simulink model "om2"  (Simulink 7.2)
settings: Solver=ode45  StartTime=0.0  StopTime=10.0  RelTol=1e-3
libraries: cdsFilt x118, cdsEpicsOut x38, cdsIPC x23, cdsMatrix x10, cdsOsc x8, cdsPhaseDeg x8, cdsEpicsIn x8, cdsRms x8, cdsProduct x5, simulink x2, cdsWD x2, cdsIPCS x1
(part 1 of 6)
settings Model: Creator=Rolf  LastModifiedBy=aivanov  ExtModeAutoUpdateStatusClock=off
settings OptimizationCC: InitFltsAndDblsToZero=on

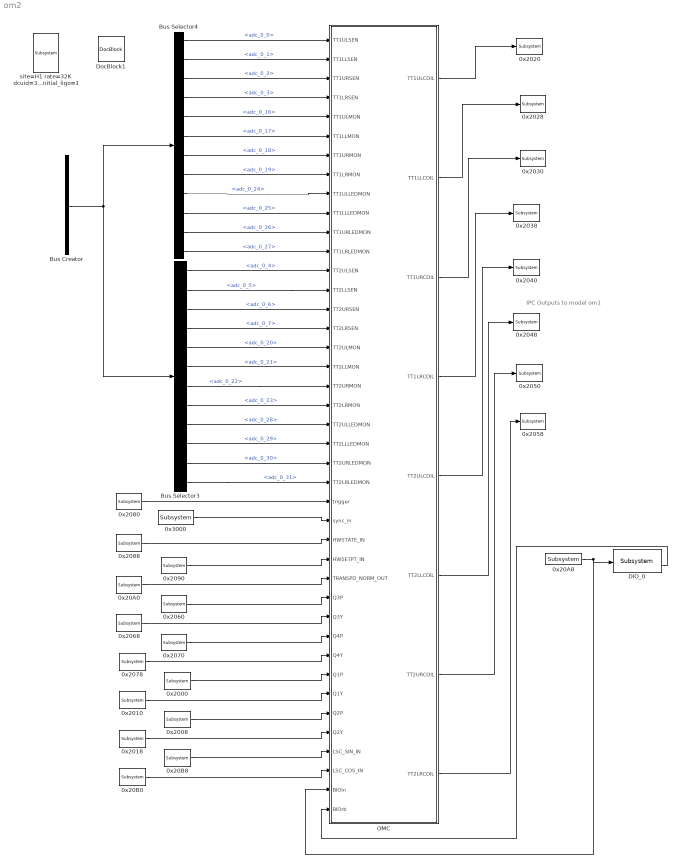
== system om2 ==
  note: IPC Outputs to model om1
  0x{2000,2008,2010,2018,2020,2028,2030,2038,2040,2048,2050,2058,2060,2068,2070,2078,2080,2088,2090} (19 alike) : cdsIPC/Subsystem  Tag=cdsIPC  Description=Inter-process communication through /rtl_epics_ipc shared memory  SystemSampleTime=-1
      settings: AttributesFormatString=%<Tag>
  0x20A0 : cdsIPC/Subsystem  Tag=cdsIPC  Description=Inter-process communication through /rtl_epics_ipc shared memory  SystemSampleTime=-1
      settings: AttributesFormatString=%<Tag>
  0x20A8 : cdsIPC/Subsystem  Tag=cdsIPC  Description=Inter-process communication through /rtl_epics_ipc shared memory  SystemSampleTime=-1
      settings: AttributesFormatString=%<Tag>
  0x20B0 : cdsIPC/Subsystem  Tag=cdsIPC  Description=Inter-process communication through /rtl_epics_ipc shared memory  SystemSampleTime=-1
      settings: AttributesFormatString=%<Tag>
  0x20B8 : cdsIPC/Subsystem  Tag=cdsIPC  Description=Inter-process communication through /rtl_epics_ipc shared memory  SystemSampleTime=-1
      settings: AttributesFormatString=%<Tag>
  0x3000 : cdsIPCS/Subsystem  Tag=cdsIPCS  SystemSampleTime=-1
      settings: AttributesFormatString=%<Tag>
  Bus Creator : BusCreator  Tag=adc_0  Description=|  Inputs='adc_0_0','adc_0_1','adc_0_2','adc_0_3','adc_0_4','adc_0_5','adc_0_6','adc_0_7','adc_0_8','adc_0_9','adc_0_10','adc_0_11','adc_0_12','adc_0_13','adc_0_14','adc_0_15','adc_0_16','adc_0_17','adc_0_18','adc_0_19','adc_0_20','adc_0_21','adc_0_22','adc_0_23','adc_0_24','adc_0_25','adc_0_26','adc_0_27','adc_0_28','adc_0_29','adc_0_30','adc_0_31'
      | PCI66-16AI64SSA
      | 40Vp-p, 16-bit, 610uV/count
      settings: AttributesFormatString=%<Description>\n%<Tag>
  Bus Selector3 : BusSelector  OutputSignals=adc_0_4,adc_0_5,adc_0_6,adc_0_7,adc_0_20,adc_0_21,adc_0_22,adc_0_23,adc_0_28,adc_0_29,adc_0_30,adc_0_31
  Bus Selector4 : BusSelector  OutputSignals=adc_0_0,adc_0_1,adc_0_2,adc_0_3,adc_0_16,adc_0_17,adc_0_18,adc_0_19,adc_0_24,adc_0_25,adc_0_26,adc_0_27
  DIO_0 : cdsRio/Subsystem  Tag=cdsRio  Description=PCI IIRO 8 relay output and isolated input module  SystemSampleTime=-1
      settings: AttributesFormatString=%<Tag>
  DocBlock1 : simulink/Model-Wide Utilities/DocBlock  Tag=SW Install  SystemSampleTime=-1  DocumentType=Text
      content=|
      | *******************************************************
      | Software installation on new computer
      | *******************************************************
      |
      | 1. Install network and PCIe cards.
      |     - Remove top cover and I/O cage.
      |     - Install NIC in PCI-X slot.
      |     - Install PCIe card for I/O chassis in PCIe slot.
      |     - Reinstall I/O cage.
      |     - Close cover.
      | 2. Connect Infiniband cables to I/O chassis and power up I/O chassis.
      | 3. Power up computer.
      | 4. Change root password.
      | 5. Modify network startup.
      |     - edit /etc/sysconfig/network-scripts (can remove all except eth0)
      |     - Change hostname in /etc/sysconfig/network file
      |     - Modify /etc/hosts
      | 6. Add users
      | 7. Make rtLinux
      |     - cd to kernel directory
      |     - Type 'make modules-install install
      |     - Edit /etc/grub_conf and change default to 0 to boot rtLinux on powerup.
      | 8. Get rid of unnecessary tasks.
      |     - cpuspeed
      |     - bluetooth
      |     - avahi daemon
      |     - cups
      |     - cups config
      |     - httpd
      |     - haldaemon
      |     - hidd
      |     - iptables
      |     - isdn
      |     - kudsu
      |     - sendmail
      |     - smartd
      |     - xfs
      | 9. reboot
      | 10. Use del key to bring up boot configuration and get rid of all unnecessary support, such as:
      |     - parallel, serial ports
      |     - USB
      | 11. Install CDS EPICS files
      |     - cd to /opt
      |     - load CDS CD (mount /dev/cdrom /mnt)
      |     - Run 'tar zxf /mnt/epics.tar.gz'
      | 12. Edit /etc/rc.local file and add:
      |     - /opt/rtlinux_dir/rtlinuxpro/mdoules/rtcore&
      |     - /opt/epics-3.14.7-linux/base/bin/linux-x86/caRepeater&
      |     - sleep 5
      |     - /etc/setup_shmem.rtl&
      | 13. Add EPICS libraries to all paths
      |     - cd to /etc/ld.so.conf.d
      |     - edit epics.conf
      |     - Add the following lines to this file:
      |         - /opt/epics-3.14.7-linux/base/lib/linux-x86
      |         - /opt/epics-3.14.7-linux/seq/lib/linux-x86
      | 14. Add CDS source code.
      |     - cd to /home/user
      |     - tar zxf /mnt/cds.tar.gz
      | 15. Build the shmem module.
      |     - cd to /home/user/cds/advLigo/src/fe/shmem
      |     - Type 'make'
      |     - cp shmem.rtl file to /etc
      | 16. Run the rc local file.
      |     - /etc/rc.local
      | 17. Create the gm files.
      |     - untar gm files in root home directory.
      |     - Type make.
      |     - Go to gm binary directory.
      |     - mkdir /opt/gm
      |     - ./GM_INSTALL
      |     - chkconfig --add gm
      |     - chkconfig gm on
      |     - service gm start
      | 18. Need to get rid of possible errors in running sequences looking for caRepeater.
      |     - ln -s /bin/true /bin/caRepeater
      | 19. Reboot
      |
      | ******* Should now be able to build FE code and EPICS.
      settings: AttributesFormatString=%<Tag>
  OMC : Subsystem  Tag=top_names
      settings: AttributesFormatString=%<Tag>
  site=H1 rate=32K dcuid=31 gds_node_id=5 no_sync=1 specific_cpu=2 compat_initial_ligo=1 : cdsParameters/Subsystem  Tag=cdsParameters  SystemSampleTime=-1
      settings: AttributesFormatString=%<Tag>
  wires:
  Bus Creator/1 -> Bus Selector4/1, Bus Selector3/1
  Bus Selector4/1 -> OMC/1(TT1ULSEN)  "<adc_0_0>"
  Bus Selector4/2 -> OMC/2(TT1LLSEN)  "<adc_0_1>"
  Bus Selector4/3 -> OMC/3(TT1URSEN)  "<adc_0_2>"
  Bus Selector4/4 -> OMC/4(TT1LRSEN)  "<adc_0_3>"
  Bus Selector4/5 -> OMC/5(TT1ULMON)  "<adc_0_16>"
  Bus Selector4/6 -> OMC/6(TT1LLMON)  "<adc_0_17>"
  Bus Selector4/7 -> OMC/7(TT1URMON)  "<adc_0_18>"
  Bus Selector4/8 -> OMC/8(TT1LRMON)  "<adc_0_19>"
  Bus Selector4/9 -> OMC/9(TT1ULLEDMON)  "<adc_0_24>"
  Bus Selector4/10 -> OMC/10(TT1LLLEDMON)  "<adc_0_25>"
  Bus Selector4/11 -> OMC/11(TT1URLEDMON)  "<adc_0_26>"
  Bus Selector4/12 -> OMC/12(TT1LRLEDMON)  "<adc_0_27>"
  Bus Selector3/1 -> OMC/13(TT2ULSEN)  "<adc_0_4>"
  Bus Selector3/2 -> OMC/14(TT2LLSEN)  "<adc_0_5>"
  Bus Selector3/4 -> OMC/16(TT2LRSEN)  "<adc_0_7>"
  Bus Selector3/5 -> OMC/17(TT2ULMON)  "<adc_0_20>"
  Bus Selector3/7 -> OMC/19(TT2URMON)  "<adc_0_22>"
  Bus Selector3/8 -> OMC/20(TT2LRMON)  "<adc_0_23>"
  Bus Selector3/9 -> OMC/21(TT2ULLEDMON)  "<adc_0_28>"
  Bus Selector3/10 -> OMC/22(TT2LLLEDMON)  "<adc_0_29>"
  Bus Selector3/11 -> OMC/23(TT2URLEDMON)  "<adc_0_30>"
  Bus Selector3/12 -> OMC/24(TT2LRLEDMON)  "<adc_0_31>"
  OMC/1(TT1ULCOIL) -> 0x2020/1
  OMC/2(TT1LLCOIL) -> 0x2028/1
  OMC/3(TT1URCOIL) -> 0x2030/1
  OMC/4(TT1LRCOIL) -> 0x2038/1
  OMC/5(TT2ULCOIL) -> 0x2040/1
  OMC/6(TT2LLCOIL) -> 0x2048/1
  OMC/7(TT2URCOIL) -> 0x2050/1
  0x2080/1 -> OMC/25(trigger)
  0x20A8/1 -> DIO_0/1, OMC/40(BIOin)
  0x2088/1 -> OMC/27(HWSTATE_IN)
  Bus Selector3/3 -> OMC/15(TT2URSEN)  "<adc_0_6>"
  0x3000/1 -> OMC/26(sync_in)
  Bus Selector3/6 -> OMC/18(TT2LLMON)  "<adc_0_21>"
  0x2090/1 -> OMC/28(HWSETPT_IN)
  0x20A0/1 -> OMC/29(TRANSPD_NORM_OUT)
  OMC/8(TT2LRCOIL) -> 0x2058/1
  0x2000/1 -> OMC/34(Q1P)
  0x2008/1 -> OMC/36(Q2P)
  0x2010/1 -> OMC/35(Q1Y)
  0x2018/1 -> OMC/37(Q2Y)
  0x2060/1 -> OMC/30(Q3P)
  0x2068/1 -> OMC/31(Q3Y)
  0x2070/1 -> OMC/32(Q4P)
  0x2078/1 -> OMC/33(Q4Y)
  0x20B8/1 -> OMC/38(LSC_SIN_IN)
  0x20B0/1 -> OMC/39(LSC_COS_IN)
  DIO_0/2 -> OMC/41(BIOrb)

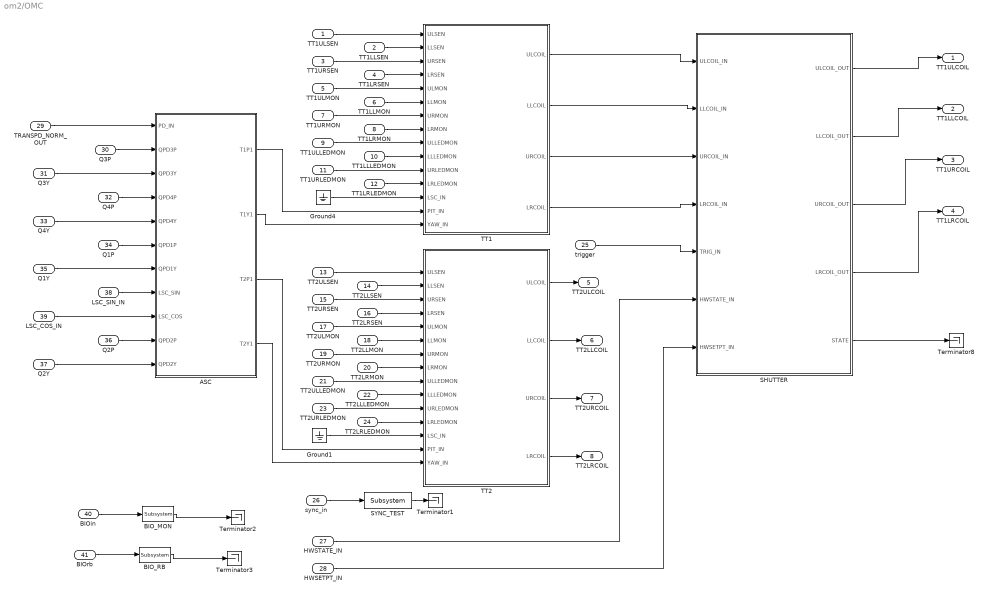
== system om2/OMC ==
  TT1ULSEN : Inport
  TT1LLSEN : Inport  Port=2
  TT1URSEN : Inport  Port=3
  TT1LRSEN : Inport  Port=4
  TT1ULMON : Inport  Port=5
  TT1LLMON : Inport  Port=6
  TT1URMON : Inport  Port=7
  TT1LRMON : Inport  Port=8
  TT1ULLEDMON : Inport  Port=9
  TT1LLLEDMON : Inport  Port=10
  TT1URLEDMON : Inport  Port=11
  TT1LRLEDMON : Inport  Port=12
  TT2ULSEN : Inport  Port=13
  TT2LLSEN : Inport  Port=14
  TT2URSEN : Inport  Port=15
  TT2LRSEN : Inport  Port=16
  TT2ULMON : Inport  Port=17
  TT2LLMON : Inport  Port=18
  TT2URMON : Inport  Port=19
  TT2LRMON : Inport  Port=20
  TT2ULLEDMON : Inport  Port=21
  TT2LLLEDMON : Inport  Port=22
  TT2URLEDMON : Inport  Port=23
  TT2LRLEDMON : Inport  Port=24
  trigger : Inport  Port=25
  sync_in : Inport  Port=26
  HWSTATE_IN : Inport  Port=27
  HWSETPT_IN : Inport  Port=28
  TRANSPD_NORM_OUT : Inport  Port=29
  Q3P : Inport  Port=30
  Q3Y : Inport  Port=31
  Q4P : Inport  Port=32
  Q4Y : Inport  Port=33
  Q1P : Inport  Port=34
  Q1Y : Inport  Port=35
  Q2P : Inport  Port=36
  Q2Y : Inport  Port=37
  LSC_SIN_IN : Inport  Port=38
  LSC_COS_IN : Inport  Port=39
  BIOin : Inport  Port=40
  BIOrb : Inport  Port=41
  ASC : Subsystem
  BIO_MON : cdsEpicsOut/Subsystem  Tag=cdsEpicsOutput  Description=|  SystemSampleTime=-1
      | Purpose:                                          
      | Output a FE signal to an EPICS channel.           
      |                                                   
      | Operation:                                        
      | Takes input value and passes it to EPICS record.  
      |                                                   
      | Usage:                                            
      | Name the part with the desired EPICS rrecord name.
      settings: AttributesFormatString=%<Tag>
  BIO_RB : cdsEpicsOut/Subsystem  Tag=cdsEpicsOutput  Description=|  SystemSampleTime=-1
      | Purpose:                                          
      | Output a FE signal to an EPICS channel.           
      |                                                   
      | Operation:                                        
      | Takes input value and passes it to EPICS record.  
      |                                                   
      | Usage:                                            
      | Name the part with the desired EPICS rrecord name.
      settings: AttributesFormatString=%<Tag>
  Ground1 : Ground
  Ground4 : Ground
  SHUTTER : Subsystem
  SYNC_TEST : cdsFilt/Subsystem  Tag=cdsFilt  Description=|  SystemSampleTime=-1
      | Purpose:                                                                                                                                                                                                                                  
      | Standard CDS IIR filter module.                                                                                                                                                                                                           
      |                                                                                                                                                                                                                                           
      | Operation:                                                                                                                                                                                                                                
      | Consists of 10 second order section IIR filters, plus a ramped gain stage. In FE code, also provides pre-defined test points and excitation channel inputs. The filter coefficients are defined in the LIGO system using the 'foton' tool.
      |                                                                                                                                                                                                                                           
      | Usage:                                                                                                                                                                                                                                    
      | Name the part with the desired filter module name.
      settings: AttributesFormatString=%<Tag>
  TT1 : Subsystem
  TT2 : Subsystem
  Terminator{1..3,8} (4 alike) : Terminator
  TT1ULCOIL : Outport  OutDataType=sfix(16)  OutScaling=2^0
  TT1LLCOIL : Outport  Port=2  OutDataType=sfix(16)  OutScaling=2^0
  TT1URCOIL : Outport  Port=3  OutDataType=sfix(16)  OutScaling=2^0
  TT1LRCOIL : Outport  Port=4  OutDataType=sfix(16)  OutScaling=2^0
  TT2ULCOIL : Outport  Port=5  OutDataType=sfix(16)  OutScaling=2^0
  TT2LLCOIL : Outport  Port=6  OutDataType=sfix(16)  OutScaling=2^0
  TT2URCOIL : Outport  Port=7  OutDataType=sfix(16)  OutScaling=2^0
  TT2LRCOIL : Outport  Port=8  OutDataType=sfix(16)  OutScaling=2^0
  wires:
  Ground1/1 -> TT2/13(LSC_IN)
  TT1/1(ULCOIL) -> SHUTTER/1(ULCOIL_IN)
  TT1/2(LLCOIL) -> SHUTTER/2(LLCOIL_IN)
  TT1/3(URCOIL) -> SHUTTER/3(URCOIL_IN)
  TT1/4(LRCOIL) -> SHUTTER/4(LRCOIL_IN)
  SHUTTER/5(STATE) -> Terminator8/1
  Ground4/1 -> TT1/13(LSC_IN)
  SHUTTER/1(ULCOIL_OUT) -> TT1ULCOIL/1
  SHUTTER/2(LLCOIL_OUT) -> TT1LLCOIL/1
  SHUTTER/3(URCOIL_OUT) -> TT1URCOIL/1
  SHUTTER/4(LRCOIL_OUT) -> TT1LRCOIL/1
  TT1ULSEN/1 -> TT1/1(ULSEN)
  TT1LLSEN/1 -> TT1/2(LLSEN)
  TT1URSEN/1 -> TT1/3(URSEN)
  TT1LRSEN/1 -> TT1/4(LRSEN)
  TT1ULMON/1 -> TT1/5(ULMON)
  TT1LLMON/1 -> TT1/6(LLMON)
  TT1URMON/1 -> TT1/7(URMON)
  TT1LRMON/1 -> TT1/8(LRMON)
  TT1ULLEDMON/1 -> TT1/9(ULLEDMON)
  TT1LLLEDMON/1 -> TT1/10(LLLEDMON)
  TT1URLEDMON/1 -> TT1/11(URLEDMON)
  TT1LRLEDMON/1 -> TT1/12(LRLEDMON)
  TT2ULSEN/1 -> TT2/1(ULSEN)
  TT2LLSEN/1 -> TT2/2(LLSEN)
  TT2URSEN/1 -> TT2/3(URSEN)
  TT2LRSEN/1 -> TT2/4(LRSEN)
  TT2ULMON/1 -> TT2/5(ULMON)
  TT2LLMON/1 -> TT2/6(LLMON)
  TT2URMON/1 -> TT2/7(URMON)
  TT2LRMON/1 -> TT2/8(LRMON)
  TT2ULLEDMON/1 -> TT2/9(ULLEDMON)
  TT2LLLEDMON/1 -> TT2/10(LLLEDMON)
  TT2URLEDMON/1 -> TT2/11(URLEDMON)
  TT2LRLEDMON/1 -> TT2/12(LRLEDMON)
  TT2/1(ULCOIL) -> TT2ULCOIL/1
  TT2/2(LLCOIL) -> TT2LLCOIL/1
  TT2/3(URCOIL) -> TT2URCOIL/1
  TT2/4(LRCOIL) -> TT2LRCOIL/1
  trigger/1 -> SHUTTER/5(TRIG_IN)
  SYNC_TEST/1 -> Terminator1/1
  sync_in/1 -> SYNC_TEST/1
  HWSTATE_IN/1 -> SHUTTER/6(HWSTATE_IN)
  HWSETPT_IN/1 -> SHUTTER/7(HWSETPT_IN)
  TRANSPD_NORM_OUT/1 -> ASC/1(PD_IN)
  ASC/1(T1P1) -> TT1/14(PIT_IN)
  ASC/2(T1Y1) -> TT1/15(YAW_IN)
  ASC/3(T2P1) -> TT2/14(PIT_IN)
  ASC/4(T2Y1) -> TT2/15(YAW_IN)
  Q3P/1 -> ASC/2(QPD3P)
  Q3Y/1 -> ASC/3(QPD3Y)
  Q4P/1 -> ASC/4(QPD4P)
  Q4Y/1 -> ASC/5(QPD4Y)
  Q1P/1 -> ASC/6(QPD1P)
  Q1Y/1 -> ASC/7(QPD1Y)
  LSC_SIN_IN/1 -> ASC/8(LSC_SIN)
  LSC_COS_IN/1 -> ASC/9(LSC_COS)
  Q2P/1 -> ASC/10(QPD2P)
  Q2Y/1 -> ASC/11(QPD2Y)
  BIO_MON/1 -> Terminator2/1
  BIOin/1 -> BIO_MON/1
  BIO_RB/1 -> Terminator3/1
  BIOrb/1 -> BIO_RB/1
